simulink model "HDLAXI4Stream"  (R2024a)
settings: Solver=FixedStepDiscrete  StartTime=0.0  StopTime=stopTime  RelTol=1e-3
values from neighbouring files (symbols this model uses):
  dataIn = [ ... (first row only)    [testAXI4Stream.m]
  fs = 100e6    (= 100000000)    [testAXI4Stream.m]
libraries: simulink x5, dspsrcs4 x2, hdlsllib x1, simulink_extras x1
settings Model: DataTypeOverride=Off  Creator=cotti  LastModifiedBy=cotti
settings OptimizationCC: BlockReduction=off  ConditionallyExecuteInputs=off  DefaultParameterBehavior=Inlined  InheritOutputTypeSmallerThanSingle=on
settings DebuggingCC: AlgebraicLoopMsg=error  SingleTaskRateTransMsg=error  UnconnectedInputMsg=warning  UnconnectedOutputMsg=warning  UnconnectedLineMsg=warning
settings HardwareCC: ProdBitPerPointer=32  ProdBitPerSizeT=32  ProdBitPerPtrDiffT=32  ProdLargestAtomicFloat=None  ProdIntDivRoundTo=Undefined  ProdEndianess=Unspecified  ProdWordSize=32  ProdHWDeviceType=ASIC/FPGA->ASIC/FPGA  TargetBitPerLong=64  TargetBitPerPointer=64  TargetBitPerSizeT=64  TargetBitPerPtrDiffT=64  TargetLongLongMode=on  TargetIntDivRoundTo=Zero  TargetEndianess=LittleEndian  TargetWordSize=64  TargetHWDeviceType=Custom Processor->MATLAB Host Computer  ProdEqTarget=off

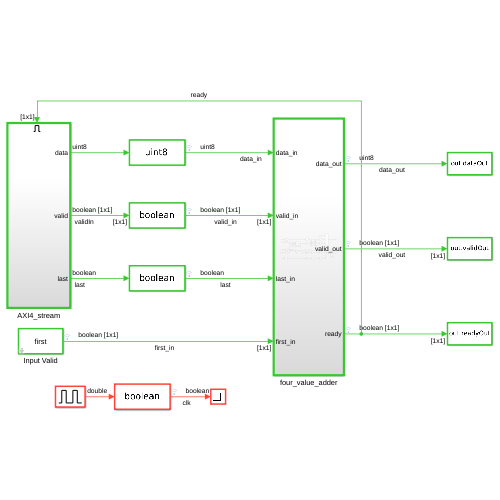
[thumbnail: Simulink's stored preview of the top-level diagram]
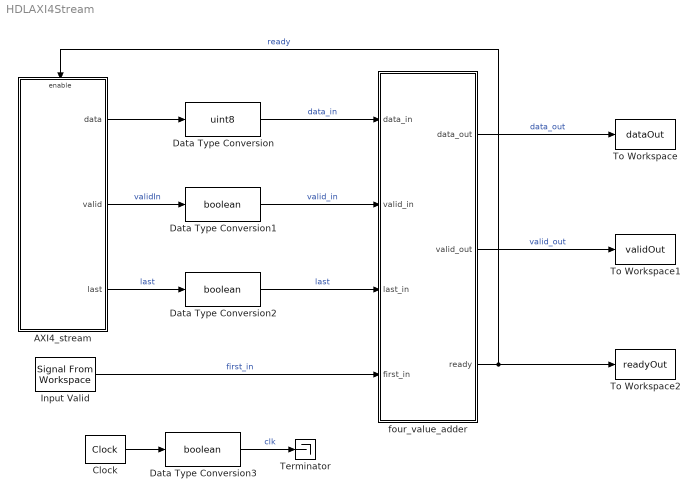
== system HDLAXI4Stream ==
  AXI4_stream : Subsystem  TreatAsAtomicUnit=on
  Clock : simulink_extras/Flip Flops/Clock  period=1/fs
  Data Type Conversion : DataTypeConversion  OutDataTypeStr=uint8  SaturateOnIntegerOverflow=off  RndMeth=Floor
  Data Type Conversion1 : DataTypeConversion  OutDataTypeStr=boolean  SaturateOnIntegerOverflow=off  RndMeth=Floor
  Data Type Conversion2 : DataTypeConversion  OutDataTypeStr=boolean  SaturateOnIntegerOverflow=off  RndMeth=Floor
  Data Type Conversion3 : DataTypeConversion  OutDataTypeStr=boolean  SaturateOnIntegerOverflow=off  RndMeth=Floor
  Input Valid : dspsrcs4/Signal From Workspace  X=first  Ts=1/fs  nsamps=1  OutputAfterFinalValue=Setting to zero  ignoreOrWarnInputAndFrameLengths=off  OutputFrames=off
  Terminator : Terminator
  To Workspace : ToWorkspace  VariableName=dataOut  SampleTime=1/fs
      settings: Save2DSignal=2-D array (concatenate along first dimension)
  To Workspace1 : ToWorkspace  VariableName=validOut  SampleTime=1/fs
      settings: Save2DSignal=2-D array (concatenate along first dimension)
  To Workspace2 : ToWorkspace  VariableName=readyOut  SampleTime=1/fs
      settings: Save2DSignal=2-D array (concatenate along first dimension)
  four_value_adder : Subsystem  TreatAsAtomicUnit=on
  wires:
  AXI4_stream/1(data) -> Data Type Conversion/1
  four_value_adder/1(data_out) -> To Workspace/1  "data_out"
  Data Type Conversion/1 -> four_value_adder/1(data_in)  "data_in"
  four_value_adder/3(ready) -> AXI4_stream/Enable, To Workspace2/1  "ready"
  AXI4_stream/2(valid) -> Data Type Conversion1/1  "validIn"
  AXI4_stream/3(last) -> Data Type Conversion2/1  "last"
  four_value_adder/2(valid_out) -> To Workspace1/1  "valid_out"
  Data Type Conversion1/1 -> four_value_adder/2(valid_in)  "valid_in"
  Data Type Conversion2/1 -> four_value_adder/3(last_in)  "last"
  Input Valid/1 -> four_value_adder/4(first_in)  "first_in"
  Clock/1 -> Data Type Conversion3/1
  Data Type Conversion3/1 -> Terminator/1  "clk"

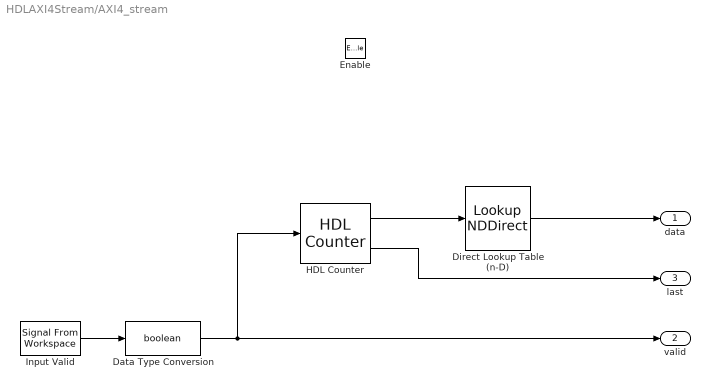
== system HDLAXI4Stream/AXI4_stream ==
  Enable : EnablePort
  Data Type Conversion : DataTypeConversion  OutDataTypeStr=boolean  SaturateOnIntegerOverflow=off  RndMeth=Floor
  Direct Lookup Table (n-D) : LookupNDDirect  NumberOfTableDimensions=1  Table=uint8(dataIn)  DiagnosticForOutOfRangeInput=Error  TableDataTypeStr=uint8
  HDL Counter : hdlsllib/Sources/HDL Counter  CountType=Count limited  CountInit=0  CountStep=1  CountMax=length(dataIn) -1  CountFromType=Initial value  CountFrom=0  CountResetPort=off  CountLoadPort=off  CountEnbPort=on  CountDirPort=off  CountHitOutputPort=on  CountDataType=Unsigned  CountWordLen=nextpow2(length(dataIn))  CountFracLen=0  CountSampTime=1
  Input Valid : dspsrcs4/Signal From Workspace  X=validIn  Ts=1/fs  nsamps=1  OutputAfterFinalValue=Setting to zero  ignoreOrWarnInputAndFrameLengths=off  OutputFrames=off
  data : Outport  InitialOutput=0  VectorParamsAs1DForOutWhenUnconnected=off
  valid : Outport  Port=2  InitialOutput=0  VectorParamsAs1DForOutWhenUnconnected=off
  last : Outport  Port=3  VectorParamsAs1DForOutWhenUnconnected=off
  wires:
  HDL Counter/1 -> Direct Lookup Table (n-D)/1
  Direct Lookup Table (n-D)/1 -> data/1
  Input Valid/1 -> Data Type Conversion/1
  Data Type Conversion/1 -> valid/1, HDL Counter/1
  HDL Counter/2 -> last/1

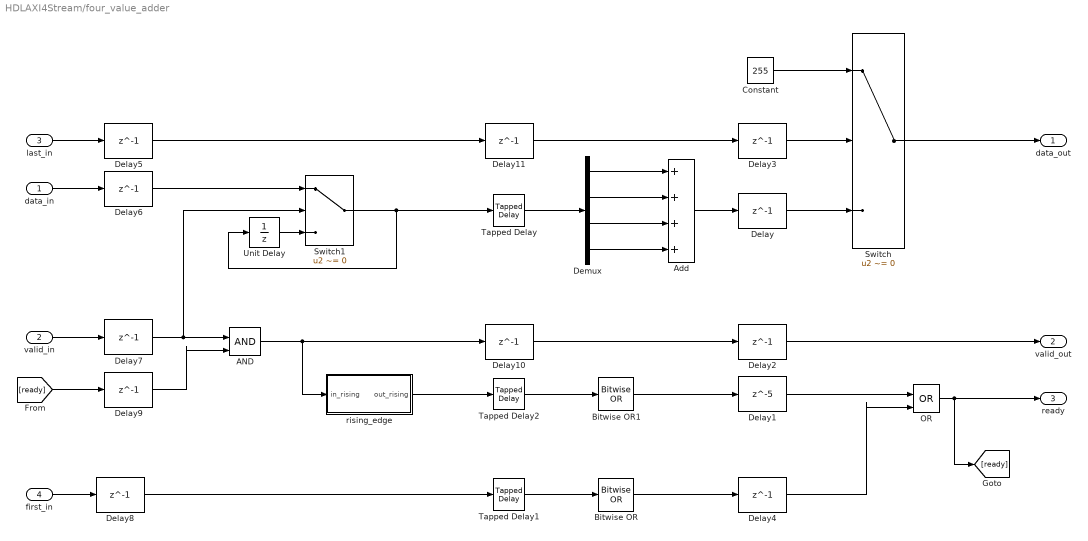
== system HDLAXI4Stream/four_value_adder ==
  data_in : Inport
  valid_in : Inport  Port=2
  last_in : Inport  Port=3
  first_in : Inport  Port=4
  AND : Logic  IconShape=distinctive  AllPortsSameDT=off  OutDataTypeStr=boolean
  Add : Sum  Inputs=++++  OutDataTypeStr=uint8
  Bitwise OR : simulink/Logic and Bit Operations/Bitwise Operator  logicop=OR  UseBitMask=off  BitMask=bin2dec('11011001')  BitMaskRealWorld=Stored Integer
      settings: LibrarySourceBlock=|
      | simulink/Quick Insert/Logic and Bit
      | Operations/Bitwise OR
  Bitwise OR1 : simulink/Logic and Bit Operations/Bitwise Operator  logicop=OR  UseBitMask=off  BitMask=bin2dec('11011001')  BitMaskRealWorld=Stored Integer
      settings: LibrarySourceBlock=|
      | simulink/Quick Insert/Logic and Bit
      | Operations/Bitwise OR
  Constant : Constant  Value=255  OutDataTypeStr=uint8  SampleTime=-1
  Delay{,2..11} (11 alike) : Delay  DelayLength=1  InitialCondition=0  UseCircularBuffer=on
  Delay1 : Delay  DelayLength=5  InitialCondition=0  UseCircularBuffer=on
  Demux : Demux
  OR : Logic  Operator=OR  IconShape=distinctive  AllPortsSameDT=off  OutDataTypeStr=boolean
  Switch : Switch  Criteria=u2 ~= 0  SaturateOnIntegerOverflow=off  InputSameDT=off
  Switch1 : Switch  Criteria=u2 ~= 0  SaturateOnIntegerOverflow=off  InputSameDT=off
  Tapped Delay : simulink/Discrete/Tapped Delay  vinit=0.0  samptime=-1  NumDelays=4  DelayOrder=Oldest  includeCurrent=off
  Tapped Delay1 : simulink/Discrete/Tapped Delay  vinit=0.0  samptime=-1  NumDelays=4  DelayOrder=Oldest  includeCurrent=off
  Tapped Delay2 : simulink/Discrete/Tapped Delay  vinit=0.0  samptime=-1  NumDelays=4  DelayOrder=Oldest  includeCurrent=off
  Unit Delay : UnitDelay  SampleTime=-1  HasFrameUpgradeWarning=on
  rising_edge : Subsystem
  data_out : Outport
  valid_out : Outport  Port=2  VectorParamsAs1DForOutWhenUnconnected=off
  ready : Outport  Port=3  VectorParamsAs1DForOutWhenUnconnected=off
  wires:
  Tapped Delay/1 -> Demux/1
  Demux/4 -> Add/4
  Demux/3 -> Add/3
  Demux/2 -> Add/2
  Demux/1 -> Add/1
  Add/1 -> Delay/1
  valid_in/1 -> Delay7/1
  Delay2/1 -> valid_out/1
  last_in/1 -> Delay5/1
  Delay/1 -> Switch/3
  Switch/1 -> data_out/1
  Constant/1 -> Switch/1
  Delay3/1 -> Switch/2
  first_in/1 -> Delay8/1
  Tapped Delay1/1 -> Bitwise OR/1
  Delay1/1 -> OR/1
  Bitwise OR/1 -> Delay4/1
  rising_edge/1(out_rising) -> Tapped Delay2/1
  Tapped Delay2/1 -> Bitwise OR1/1
  Bitwise OR1/1 -> Delay1/1
  Delay4/1 -> OR/2
  Delay8/1 -> Tapped Delay1/1
  [ready] -> Delay9/1
  Delay7/1 -> Switch1/2, AND/1
  AND/1 -> rising_edge/1(in_rising), Delay10/1
  Delay9/1 -> AND/2
  Delay10/1 -> Delay2/1
  Delay11/1 -> Delay3/1
  OR/1 -> [ready], ready/1
  Delay6/1 -> Switch1/1
  Unit Delay/1 -> Switch1/3
  Switch1/1 -> Tapped Delay/1, Unit Delay/1
  data_in/1 -> Delay6/1
  Delay5/1 -> Delay11/1

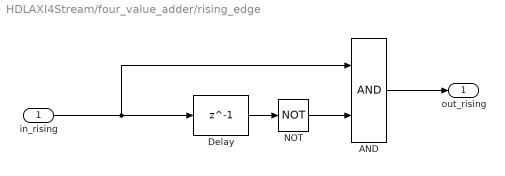
== system HDLAXI4Stream/four_value_adder/rising_edge ==
  in_rising : Inport
  AND : Logic  IconShape=distinctive  AllPortsSameDT=off  OutDataTypeStr=boolean
  Delay : Delay  DelayLength=1  InitialCondition=0  UseCircularBuffer=on
  NOT : Logic  Operator=NOT  IconShape=distinctive  AllPortsSameDT=off  OutDataTypeStr=boolean
  out_rising : Outport
  wires:
  in_rising/1 -> AND/1, Delay/1
  AND/1 -> out_rising/1
  Delay/1 -> NOT/1
  NOT/1 -> AND/2
